simulink model "IF_Subsystem"  (R2024b)
settings: Solver=FixedStepAuto  StartTime=0.0  StopTime=20  FixedStep=0.001  RelTol=1e-3
libraries: simulink x2, spsSawtoothGeneratorLib x1
settings Model: Creator=abdal  LastModifiedBy=abdal

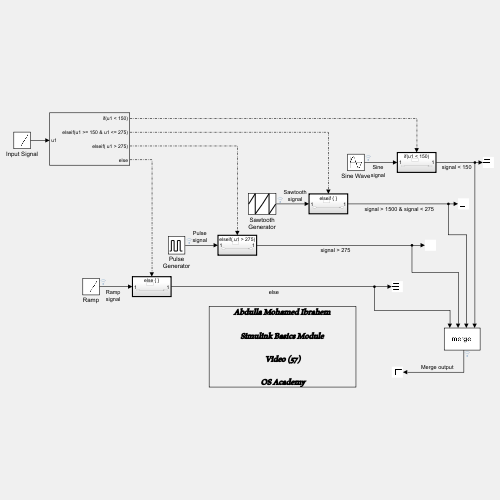
[thumbnail: Simulink's stored preview of the top-level diagram]
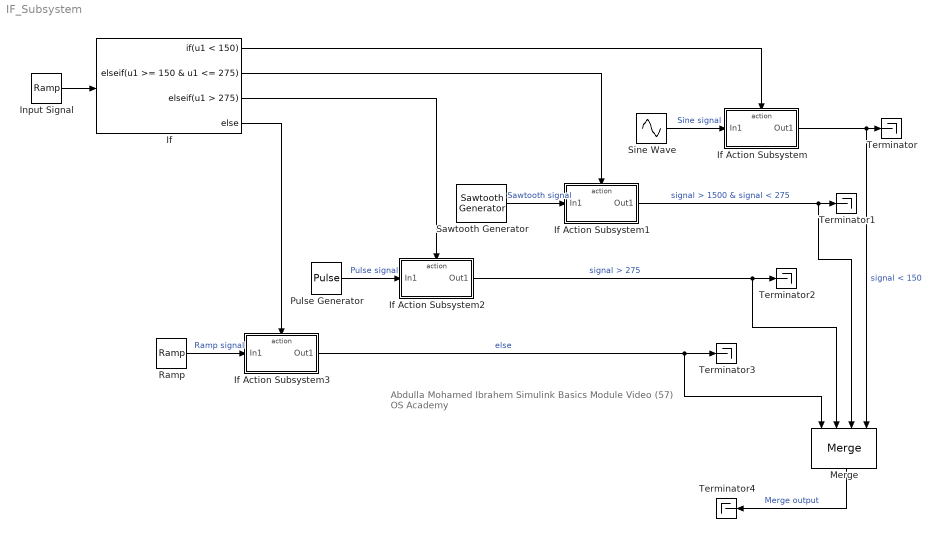
== system IF_Subsystem ==
  note: Abdulla Mohamed Ibrahem
      | Simulink Basics Module
      | Video (57)
      | OS Academy
  If : If  IfExpression=u1 < 150  ElseIfExpressions=u1 >= 150 & u1 <= 275, u1 > 275
  If Action Subsystem : Subsystem  TreatAsAtomicUnit=on
  If Action Subsystem1 : Subsystem  TreatAsAtomicUnit=on
  If Action Subsystem2 : Subsystem  TreatAsAtomicUnit=on
  If Action Subsystem3 : Subsystem  TreatAsAtomicUnit=on
  Input Signal : simulink/Sources/Ramp  slope=20  start=2  InitialOutput=-10
  Merge : Merge  Inputs=4
  Pulse Generator : DiscretePulseGenerator  PulseType=Time based  Period=1  PulseWidth=50
  Ramp : simulink/Sources/Ramp  slope=2  start=1  InitialOutput=-3
  Sawtooth Generator : spsSawtoothGeneratorLib/Sawtooth Generator  Freq=0.5  Phase=180  Ts=0
  Sine Wave : Sin  SampleTime=0
  Terminator{,1..4} (5 alike) : Terminator
  wires:
  Input Signal/1 -> If/1
  If/1 -> If Action Subsystem/Action
  If/2 -> If Action Subsystem1/Action
  If/3 -> If Action Subsystem2/Action
  If/4 -> If Action Subsystem3/Action
  If Action Subsystem/1(Out1) -> Merge/4, Terminator/1  "signal < 150"
  If Action Subsystem1/1(Out1) -> Terminator1/1, Merge/3  "signal > 1500 & signal < 275"
  If Action Subsystem2/1(Out1) -> Merge/2, Terminator2/1  "signal > 275"
  If Action Subsystem3/1(Out1) -> Merge/1, Terminator3/1  "else"
  Merge/1 -> Terminator4/1  "Merge output"
  Sine Wave/1 -> If Action Subsystem/1(In1)  "Sine signal"
  Sawtooth Generator/1 -> If Action Subsystem1/1(In1)  "Sawtooth signal"
  Ramp/1 -> If Action Subsystem3/1(In1)  "Ramp signal"
  Pulse Generator/1 -> If Action Subsystem2/1(In1)  "Pulse signal"

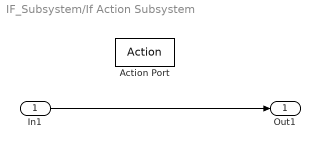
== system IF_Subsystem/If Action Subsystem ==
  In1 : Inport
  Action Port : ActionPort  ActionPortLabel=if(u1 < 150)
  Out1 : Outport
  wires:
  In1/1 -> Out1/1

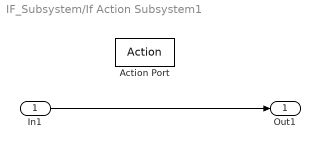
== system IF_Subsystem/If Action Subsystem1 ==
  In1 : Inport
  Action Port : ActionPort  ActionPortLabel=elseif(u1 >= 150 & u1 <= 275)
  Out1 : Outport
  wires:
  In1/1 -> Out1/1

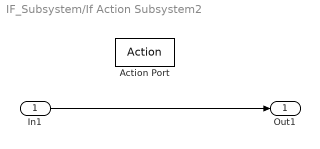
== system IF_Subsystem/If Action Subsystem2 ==
  In1 : Inport
  Action Port : ActionPort  ActionPortLabel=elseif( u1 > 275)
  Out1 : Outport
  wires:
  In1/1 -> Out1/1

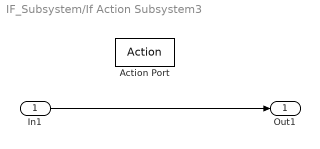
== system IF_Subsystem/If Action Subsystem3 ==
  In1 : Inport
  Action Port : ActionPort  ActionPortLabel=else
  Out1 : Outport
  wires:
  In1/1 -> Out1/1
